simulink model "Project1"  (R2023a)
settings: Solver=VariableStepAuto  StartTime=0.0  StopTime=10.0  RelTol=1e-3
settings Model: Creator=HP  LastModifiedBy=HP

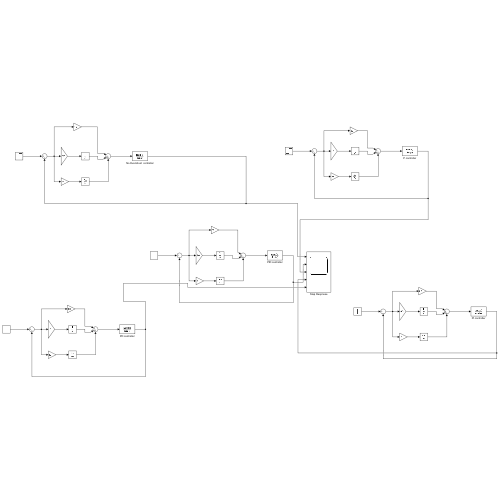
[thumbnail: Simulink's stored preview of the top-level diagram]
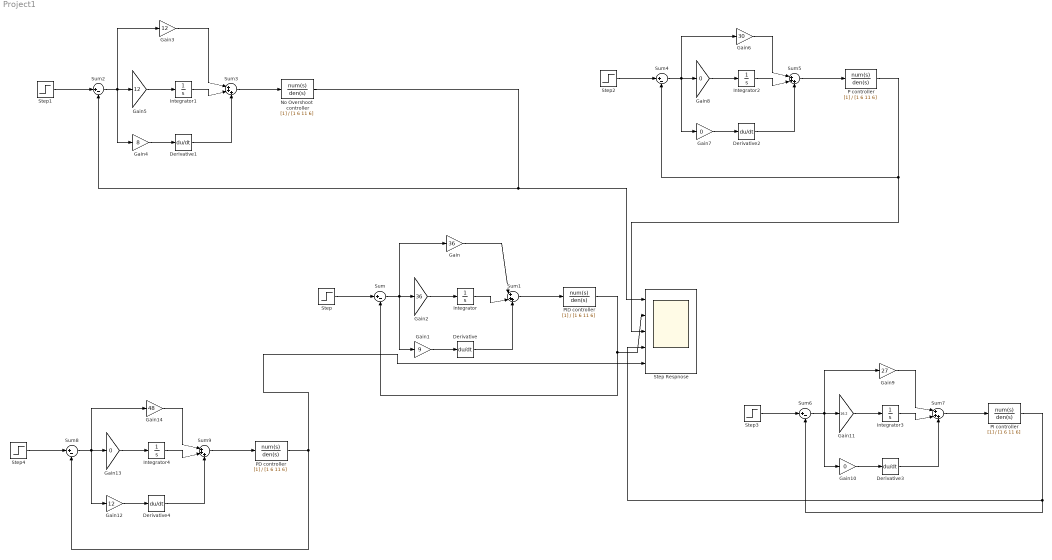
== system Project1 ==
  Derivative{,1..4} (5 alike) : Derivative
  Gain : Gain  Gain=36
  Gain1 : Gain  Gain=9
  Gain{7..8,10,13} (4 alike) : Gain  Gain=0
  Gain11 : Gain  Gain=16.2
  Gain12 : Gain  Gain=12
  Gain14 : Gain  Gain=48
  Gain2 : Gain  Gain=36
  Gain3 : Gain  Gain=12
  Gain4 : Gain  Gain=8
  Gain5 : Gain  Gain=12
  Gain6 : Gain  Gain=30
  Gain9 : Gain  Gain=27
  Integrator{,1..4} (5 alike) : Integrator
  No Overshoot  controller : TransferFcn  Denominator=[1 6 11 6]
  P controller : TransferFcn  Denominator=[1 6 11 6]
  PD controller : TransferFcn  Denominator=[1 6 11 6]
  PI controller : TransferFcn  Denominator=[1 6 11 6]
  PID controller : TransferFcn  Denominator=[1 6 11 6]
  Step{,1..4} (5 alike) : Step  SampleTime=0
  Step Respnose : Scope  NumInputPorts=5
  Sum{,2,4,6,8} (5 alike) : Sum  Inputs=|+-
  Sum{1,3,5,7,9} (5 alike) : Sum  Inputs=|+++
  wires:
  Step/1 -> Sum/1
  Sum/1 -> Gain1/1, Gain2/1, Gain/1
  Sum1/1 -> PID controller/1
  PID controller/1 -> Sum/2, Step Respnose/2
  Gain1/1 -> Derivative/1
  Gain2/1 -> Integrator/1
  Derivative/1 -> Sum1/3
  Integrator/1 -> Sum1/2
  Gain/1 -> Sum1/1
  Derivative1/1 -> Sum3/3
  Gain3/1 -> Sum3/1
  Integrator1/1 -> Sum3/2
  Gain5/1 -> Integrator1/1
  No Overshoot  controller/1 -> Step Respnose/1, Sum2/2
  Step1/1 -> Sum2/1
  Sum2/1 -> Gain4/1, Gain5/1, Gain3/1
  Gain4/1 -> Derivative1/1
  Sum3/1 -> No Overshoot  controller/1
  Derivative2/1 -> Sum5/3
  Gain6/1 -> Sum5/1
  Integrator2/1 -> Sum5/2
  Gain8/1 -> Integrator2/1
  P controller/1 -> Step Respnose/3, Sum4/2
  Step2/1 -> Sum4/1
  Sum4/1 -> Gain7/1, Gain8/1, Gain6/1
  Gain7/1 -> Derivative2/1
  Sum5/1 -> P controller/1
  Derivative3/1 -> Sum7/3
  Gain9/1 -> Sum7/1
  Integrator3/1 -> Sum7/2
  Gain11/1 -> Integrator3/1
  PI controller/1 -> Step Respnose/4, Sum6/2
  Step3/1 -> Sum6/1
  Sum6/1 -> Gain10/1, Gain11/1, Gain9/1
  Gain10/1 -> Derivative3/1
  Sum7/1 -> PI controller/1
  Gain12/1 -> Derivative4/1
  PD controller/1 -> Sum8/2, Step Respnose/5
  Gain13/1 -> Integrator4/1
  Integrator4/1 -> Sum9/2
  Gain14/1 -> Sum9/1
  Sum8/1 -> Gain12/1, Gain13/1, Gain14/1
  Derivative4/1 -> Sum9/3
  Step4/1 -> Sum8/1
  Sum9/1 -> PD controller/1
